simulink model "ecm_ekf"  (R2026a)
settings: Solver=FixedStepDiscrete  FixedStep=1
values from neighbouring files (symbols this model uses):
  docvCoeffs_ws = ocvModel.derivativeCoefficients    [runSimulinkValidation.m]
  ocvCoeffs_ws = ocvModel.coefficients    [runSimulinkValidation.m]
settings Model: Creator=valio  LastModifiedBy=valio

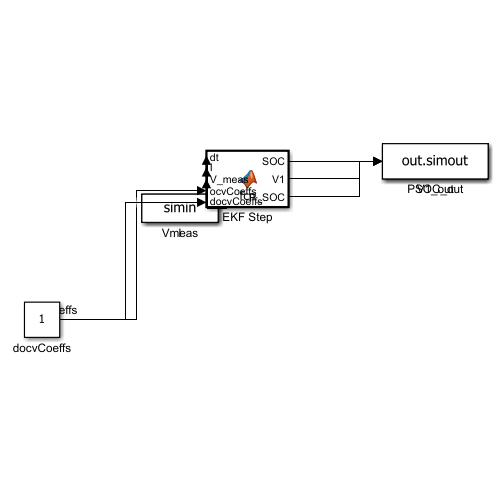
[thumbnail: Simulink's stored preview of the top-level diagram]
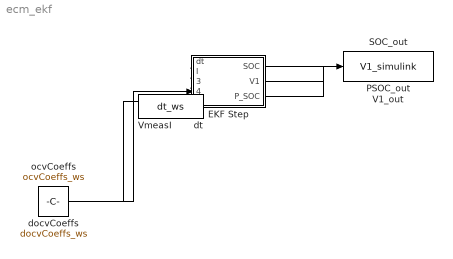
== system ecm_ekf ==
  EKF Step : MATLAB Function  TreatAsAtomicUnit=on
  I : FromWorkspace  VariableName=I_ws  SampleTime=1  ZeroCross=off
  PSOC_out : ToWorkspace  VariableName=PSOC_simulink  SampleTime=-1
  SOC_out : ToWorkspace  VariableName=SOC_simulink  SampleTime=-1
  V1_out : ToWorkspace  VariableName=V1_simulink  SampleTime=-1
  Vmeas : FromWorkspace  VariableName=V_ws  SampleTime=1  ZeroCross=off
  docvCoeffs : Constant  Value=docvCoeffs_ws
  dt : FromWorkspace  VariableName=dt_ws  SampleTime=1  ZeroCross=off
  ocvCoeffs : Constant  Value=ocvCoeffs_ws
  wires:
  dt/1 -> EKF Step/1(dt)
  I/1 -> EKF Step/2(I)
  Vmeas/1 -> EKF Step/3(V_meas)
  ocvCoeffs/1 -> EKF Step/4(ocvCoeffs)
  docvCoeffs/1 -> EKF Step/5(docvCoeffs)
  EKF Step/1(SOC) -> SOC_out/1
  EKF Step/2(V1) -> V1_out/1
  EKF Step/3(P_SOC) -> PSOC_out/1

== matlab function ecm_ekf/EKF Step ==
  data: dt input; SOC output; I input; V_meas input; ocvCoeffs input; docvCoeffs input; V1 output; P_SOC output
function [SOC, V1, P_SOC] = ekfStep(dt, I, V_meas, ocvCoeffs, docvCoeffs)
%#codegen
% One predict+update step. Persistent state holds [SOC;V1] and P
% between calls, mirroring the running x/P in ekfEstimate.m's
% for-loop. dt==0 on the first call (see runSimulinkValidation.m,
% dt_ws(1,2)=0) is the init trigger - same as ekfEstimate.m's k=1
% special case, no predict/update on that first sample.

persistent x P;

% Hardcoded to match experiments/expA_nominal.m.
% For Experiments B-E, change SOC0/R0/R1/tau/Q_As/tuning here to
% match that experiment's script - nothing else needs to change.
SOC0  = 1.0;
R0    = 0.0312244650416;
R1    = 0.0113287933401;
tau   = 5.23962539484;
Q_As  = 2.997393193 * 3600;
P0_SOC = (0.01)^2; P0_V1 = (0.01)^2;
q_SOC  = 1e-10;    q_V1  = 1e-6;
R_V    = (3e-3)^2;

if isempty(x)
    x = [SOC0; 0];
    P = diag([P0_SOC, P0_V1]);
end

if dt > 0
    alpha = exp(-dt / tau);
    x_pred = [x(1) - (dt / Q_As) * I; ...
        alpha * x(2) + (1 - alpha) * R1 * I];
    F = [1, 0; 0, alpha];
    Qk = diag([q_SOC, q_V1]);
    P_pred = F * P * F.' + Qk;

    ocv_V = polyval(ocvCoeffs, x_pred(1));
    docv_V = polyval(docvCoeffs, x_pred(1));
    y_pred = ocv_V - x_pred(2) - R0 * I;
    resid = V_meas - y_pred;

    H = [docv_V, -1];
    S = H * P_pred * H.' + R_V;
    K = (P_pred * H.') / S;

    x_upd = x_pred + K * resid;
    P_upd = (eye(2) - K * H) * P_pred;
    x_upd(1) = min(max(x_upd(1), 0), 1);

    x = x_upd;
    P = P_upd;
end

SOC = x(1);
V1 = x(2);
P_SOC = P(1, 1);
end
